simulink library "Fuel"  (Simulink 8.2)
settings: Solver=ode45  StartTime=0.0  StopTime=10.0  RelTol=1e-3
settings Model: Creator=lena.frank  LastModifiedBy=drhf

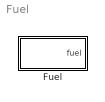
== system Fuel ==
  Fuel : Subsystem  mask(fuel_source){ft=1, t=20, ls=3.5, p=1.013e5, h_values=[5.14e7 5.69e7], tc=45, price=1, mass=[0.33 0.67 0 0 0 0]}
      mask prompts: ft "fuel (0=no calculation; 1=gaseous; 2=liquid; 3=solid)"; t "temperature [°C]"; ls "stoichiometric air demand [kg/kg]"; p "pressure [Pa]"; h_values "heat without/with condensation [J/kg]"; tc "condensation temperature [°C]"; price "price of fuel per kg [arb. unit]"; mass "massfraction [H C O S N H2O] [-]"
      mask Help: web(fullfile(path_carnot('help'),'Fuel.html'),'-helpbrowser')

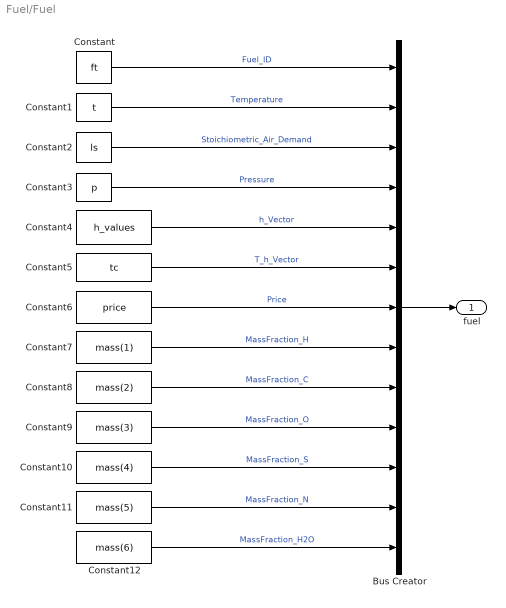
== system Fuel/Fuel ==
  Bus Creator : BusCreator  Inputs=13
  Constant : Constant  Value=ft
  Constant1 : Constant  Value=t
  Constant10 : Constant  Value=mass(4)
  Constant11 : Constant  Value=mass(5)
  Constant12 : Constant  Value=mass(6)
  Constant2 : Constant  Value=ls
  Constant3 : Constant  Value=p
  Constant4 : Constant  Value=h_values
  Constant5 : Constant  Value=tc
  Constant6 : Constant  Value=price
  Constant7 : Constant  Value=mass(1)
  Constant8 : Constant  Value=mass(2)
  Constant9 : Constant  Value=mass(3)
  fuel : Outport  InitialOutput=0
  wires:
  Constant/1 -> Bus Creator/1  "Fuel_ID"
  Constant1/1 -> Bus Creator/2  "Temperature"
  Constant2/1 -> Bus Creator/3  "Stoichiometric_Air_Demand"
  Constant3/1 -> Bus Creator/4  "Pressure"
  Constant4/1 -> Bus Creator/5  "h_Vector"
  Constant5/1 -> Bus Creator/6  "T_h_Vector"
  Constant6/1 -> Bus Creator/7  "Price"
  Constant7/1 -> Bus Creator/8  "MassFraction_H"
  Bus Creator/1 -> fuel/1
  Constant8/1 -> Bus Creator/9  "MassFraction_C"
  Constant9/1 -> Bus Creator/10  "MassFraction_O"
  Constant10/1 -> Bus Creator/11  "MassFraction_S"
  Constant11/1 -> Bus Creator/12  "MassFraction_N"
  Constant12/1 -> Bus Creator/13  "MassFraction_H2O"
